simulink model "TCS1"  (R2024b)
settings: Solver=ode45  StartTime=0.0  StopTime=20  RelTol=1e-3
InitFcn:
  | Cte_TP_ABS_CHERIF
values from neighbouring files (symbols this model uses):
  g = 9.81    [Cte_TP_ABS_CHERIF.m]    (also in Cte_Traction.m)
  m = 1000    [Cte_TP_ABS_CHERIF.m]    (also in Cte_Traction.m = 1500)
  rRoue = 0.3    [Cte_TP_ABS_CHERIF.m]
libraries: simulink x4
settings Model: Creator=enzoc  LastModifiedBy=enzoc
settings SolverCC: ZeroCrossAlgorithm=Adaptive
settings DebuggingCC: IgnoredZcDiagnostic=none

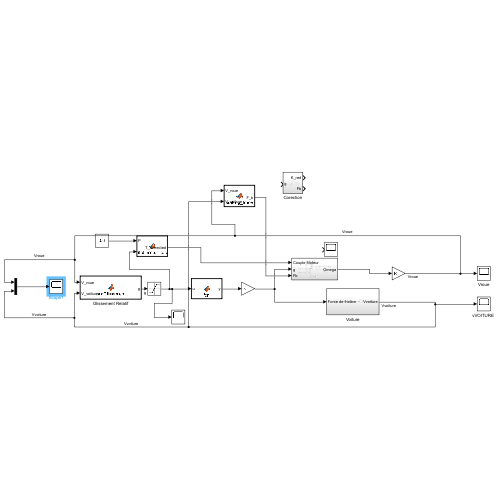
[thumbnail: Simulink's stored preview of the top-level diagram]
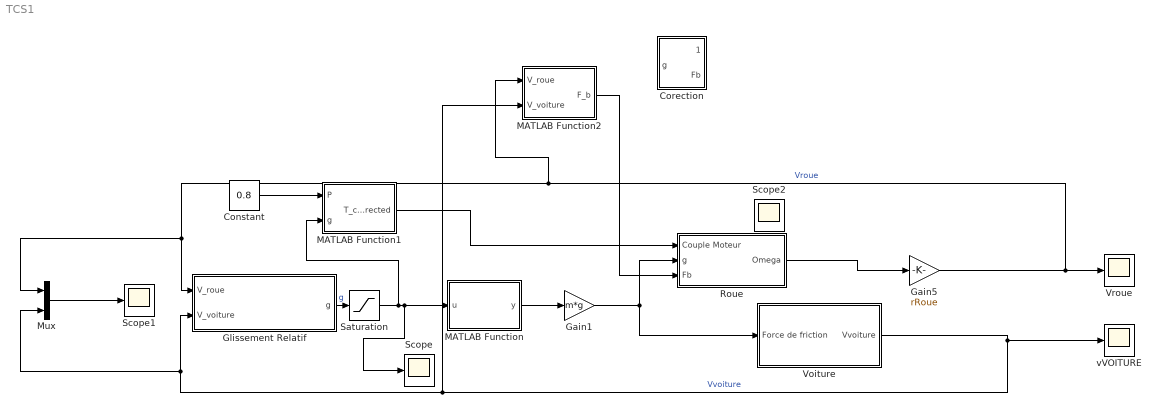
== system TCS1 ==
  Constant : Constant  Value=0.8
  Corection : Subsystem
  Gain1 : Gain  Gain=m*g
  Gain5 : Gain  Gain=rRoue
  Glissement Relatif : MATLAB Function  TreatAsAtomicUnit=on
  MATLAB Function : MATLAB Function  TreatAsAtomicUnit=on
  MATLAB Function1 : MATLAB Function  TreatAsAtomicUnit=on
  MATLAB Function2 : MATLAB Function  TreatAsAtomicUnit=on
  Mux : Mux  Inputs=2
  Roue : Subsystem
  Saturation : Saturate  UpperLimit=1  LowerLimit=-1
  Scope : Scope
  Scope1 : Scope
  Scope2 : Scope
  Voiture : Subsystem
  Vroue : Scope
  "vVOITURE " : Scope
  wires:
  Gain5/1 -> Mux/1, Glissement Relatif/1(V_roue), MATLAB Function2/1(V_roue), Vroue/1  "Vroue"
  Roue/1(Omega) -> Gain5/1
  Voiture/1(Vvoiture) -> MATLAB Function2/2(V_voiture), Mux/2, Glissement Relatif/2(V_voiture), "vVOITURE "/1  "Vvoiture"
  Mux/1 -> Scope1/1
  MATLAB Function/1(y) -> Gain1/1
  Glissement Relatif/1(g) -> Saturation/1  "g"
  Saturation/1 -> MATLAB Function1/2(g), MATLAB Function/1(u), Scope/1
  Gain1/1 -> Roue/2(g), Voiture/1(Force de friction)
  MATLAB Function2/1(F_b) -> Roue/3(Fb)
  MATLAB Function1/1(T_corrected) -> Roue/1(Couple Moteur)
  Constant/1 -> MATLAB Function1/1(P)

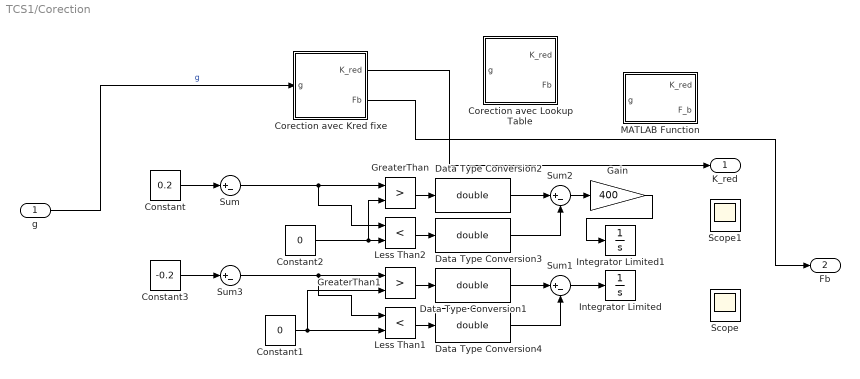
== system TCS1/Corection ==
  g : Inport
  Constant : Constant  Value=0.2
  Constant1 : Constant  Value=0
  Constant2 : Constant  Value=0
  Constant3 : Constant  Value=-0.2
  Corection avec Kred fixe : Subsystem
  Corection avec Lookup Table : Subsystem
  Data Type Conversion{1..4} (4 alike) : DataTypeConversion  OutDataTypeStr=double  SaturateOnIntegerOverflow=off
  Gain : Gain  Gain=400
  GreaterThan : RelationalOperator  Operator=>  OutDataTypeStr=boolean  RndMeth=Simplest  InputSameDT=off
  GreaterThan1 : RelationalOperator  Operator=>  OutDataTypeStr=boolean  RndMeth=Simplest  InputSameDT=off
  Integrator Limited : Integrator  LimitOutput=on  UpperSaturationLimit=1  LowerSaturationLimit=0
  Integrator Limited1 : Integrator  LimitOutput=on  UpperSaturationLimit=1  LowerSaturationLimit=0
  Less Than1 : RelationalOperator  Operator=<  OutDataTypeStr=boolean  RndMeth=Simplest  InputSameDT=off
  Less Than2 : RelationalOperator  Operator=<  OutDataTypeStr=boolean  RndMeth=Simplest  InputSameDT=off
  MATLAB Function : MATLAB Function  TreatAsAtomicUnit=on
  Scope : Scope
  Scope1 : Scope
  Sum{,1..3} (4 alike) : Sum  Inputs=|+-
  K_red : Outport
  Fb : Outport  Port=2
  wires:
  Constant/1 -> Sum/1
  Constant2/1 -> Less Than2/2, GreaterThan/2
  GreaterThan/1 -> Data Type Conversion2/1
  Sum2/1 -> Gain/1
  Data Type Conversion3/1 -> Sum2/2
  Sum/1 -> GreaterThan/1, Less Than2/1
  Less Than2/1 -> Data Type Conversion3/1
  Data Type Conversion2/1 -> Sum2/1
  Gain/1 -> Integrator Limited1/1
  Sum3/1 -> GreaterThan1/1, Less Than1/1
  Constant1/1 -> Less Than1/2, GreaterThan1/2
  Less Than1/1 -> Data Type Conversion4/1
  Data Type Conversion4/1 -> Sum1/2
  GreaterThan1/1 -> Data Type Conversion1/1
  Data Type Conversion1/1 -> Sum1/1
  Constant3/1 -> Sum3/1
  Sum1/1 -> Integrator Limited/1
  Corection avec Kred fixe/2(Fb) -> Fb/1
  Corection avec Kred fixe/1(K_red) -> K_red/1
  g/1 -> Corection avec Kred fixe/1(g)  "g"

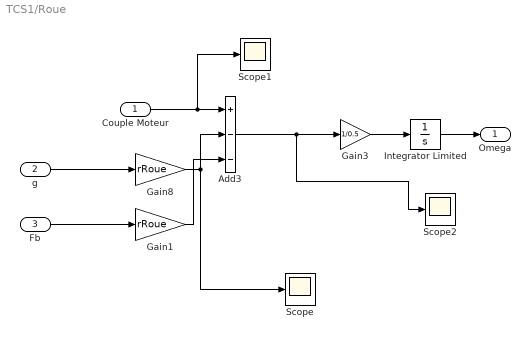
== system TCS1/Roue ==
  Couple Moteur : Inport
  g : Inport  Port=2
  Fb : Inport  Port=3
  Add3 : Sum  Inputs=+--
  Gain1 : Gain  Gain=rRoue
  Gain3 : Gain  Gain=1/0.5
  Gain8 : Gain  Gain=rRoue
  Integrator Limited : Integrator  LimitOutput=on  UpperSaturationLimit=1000  LowerSaturationLimit=0
  Scope : Scope
  Scope1 : Scope
  Scope2 : Scope
  Omega : Outport
  wires:
  Couple Moteur/1 -> Scope1/1, Add3/1
  g/1 -> Gain8/1
  Gain8/1 -> Scope/1, Add3/2
  Add3/1 -> Scope2/1, Gain3/1
  Gain3/1 -> Integrator Limited/1
  Integrator Limited/1 -> Omega/1
  Fb/1 -> Gain1/1
  Gain1/1 -> Add3/3

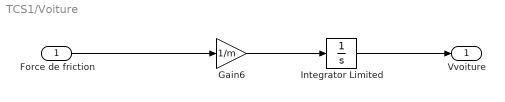
== system TCS1/Voiture ==
  Force de friction : Inport
  Gain6 : Gain  Gain=1/m
  Integrator Limited : Integrator  LimitOutput=on  UpperSaturationLimit=+inf  LowerSaturationLimit=0
  Vvoiture : Outport
  wires:
  Gain6/1 -> Integrator Limited/1
  Integrator Limited/1 -> Vvoiture/1
  Force de friction/1 -> Gain6/1

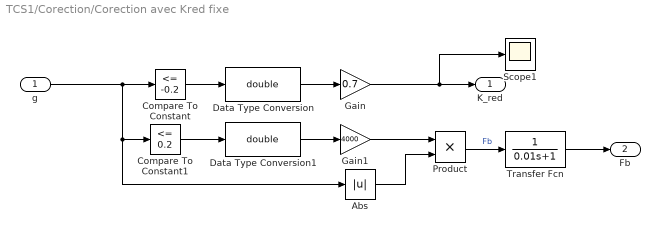
== system TCS1/Corection/Corection avec Kred fixe ==
  g : Inport
  Abs : Abs  SaturateOnIntegerOverflow=off
  Compare To Constant : simulink/Logic and Bit Operations/Compare To Constant  relop=<=  const=-0.2  OutDataTypeStr=boolean
  Compare To Constant1 : simulink/Logic and Bit Operations/Compare To Constant  relop=<=  const=0.2  OutDataTypeStr=boolean
  Data Type Conversion : DataTypeConversion  OutDataTypeStr=double  SaturateOnIntegerOverflow=off  RndMeth=Floor
  Data Type Conversion1 : DataTypeConversion  OutDataTypeStr=double  SaturateOnIntegerOverflow=off  RndMeth=Floor
  Gain : Gain  Gain=0.7
  Gain1 : Gain  Gain=4000
  Product : Product
  Scope1 : Scope
  Transfer Fcn : TransferFcn  Denominator=[0.01 1]
  K_red : Outport
  Fb : Outport  Port=2
  wires:
  g/1 -> Abs/1, Compare To Constant1/1, Compare To Constant/1
  Product/1 -> Transfer Fcn/1  "Fb"
  Abs/1 -> Product/2
  Data Type Conversion1/1 -> Gain1/1
  Compare To Constant/1 -> Data Type Conversion/1
  Compare To Constant1/1 -> Data Type Conversion1/1
  Gain1/1 -> Product/1
  Transfer Fcn/1 -> Fb/1
  Data Type Conversion/1 -> Gain/1
  Gain/1 -> Scope1/1, K_red/1

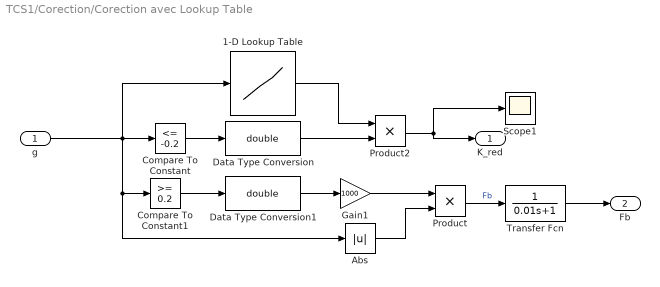
== system TCS1/Corection/Corection avec Lookup Table ==
  g : Inport
  1-D Lookup Table : Lookup_n-D  NumberOfTableDimensions=1  BreakpointsForDimension1=[-1.0, -0.9, -0.8, -0.7, -0.6, -0.5, -0.4, -0.3, -0.2, 0]  Table=[0.1, 0.15, 0.25, 0.35, 0.45, 0.55, 0.65, 0.75, 0.85, 1.0]  InternalRulePriority=Speed  RndMeth=Simplest
  Abs : Abs  SaturateOnIntegerOverflow=off
  Compare To Constant : simulink/Logic and Bit Operations/Compare To Constant  relop=<=  const=-0.2  OutDataTypeStr=boolean
  Compare To Constant1 : simulink/Logic and Bit Operations/Compare To Constant  relop=>=  const=0.2  OutDataTypeStr=boolean
  Data Type Conversion : DataTypeConversion  OutDataTypeStr=double  SaturateOnIntegerOverflow=off  RndMeth=Floor
  Data Type Conversion1 : DataTypeConversion  OutDataTypeStr=double  SaturateOnIntegerOverflow=off  RndMeth=Floor
  Gain1 : Gain  Gain=1000
  Product : Product
  Product2 : Product
  Scope1 : Scope
  Transfer Fcn : TransferFcn  Denominator=[0.01 1]
  K_red : Outport
  Fb : Outport  Port=2
  wires:
  g/1 -> 1-D Lookup Table/1, Abs/1, Compare To Constant1/1, Compare To Constant/1
  Product/1 -> Transfer Fcn/1  "Fb"
  Abs/1 -> Product/2
  Data Type Conversion1/1 -> Gain1/1
  Compare To Constant/1 -> Data Type Conversion/1
  Compare To Constant1/1 -> Data Type Conversion1/1
  Data Type Conversion/1 -> Product2/2
  Gain1/1 -> Product/1
  1-D Lookup Table/1 -> Product2/1
  Product2/1 -> K_red/1, Scope1/1
  Transfer Fcn/1 -> Fb/1

== matlab function TCS1/Corection/MATLAB Function ==
  data: g input; K_red output; F_b output
function [K_red, F_b] = traction_control(g)
    % Paramètres
    g_seuil_haut = 0.2;  % Seuil supérieur de glissement
    g_seuil_bas = -0.2;  % Seuil inférieur de glissement
    K_frein = 1000;      % Gain pour la force de freinage
    
    % Lookup Table pour K_red
    g_points = [-1, -0.9, -0.8, -0.7, -0.6, -0.5, -0.4, -0.3, -0.2, 0];
    K_red_points = [0.1, 0.15, 0.25, 0.35, 0.45, 0.55, 0.65, 0.75, 0.85, 1.0];
    
    % Initialisation des sorties
    K_red = 1.0;  % Par défaut, pas de réduction
    F_b = 0;      % Pas de freinage par défaut
    
    % Logique de contrôle pour K_red
    if g <= g_seuil_bas
        % Interpolation pour K_red en fonction de g
        K_red = interp1(g_points, K_red_points, g, 'linear', 'extrap');
    end
    
    % Logique de contrôle pour F_b
    if g > g_seuil_haut
        % Appliquer un freinage proportionnel au glissement positif excessif
        F_b = K_frein * abs(g);
    end
end

== matlab function TCS1/MATLAB Function ==
  data: u input; y output
function y = fcn(u)

y = u;

== matlab function TCS1/MATLAB Function1 ==
  data: P input; T_corrected output; g input
function T_corrected = correct_motor_torque(P, g)
    % Function to correct the motor torque based on pedal input and slip ratio
    % All parameters are defined internally.
    %
    % Inputs:
    %   P - Pedal position (0 to 1)
    %   g - Current slip ratio (dimensionless)
    %
    % Output:
    %   T_corrected - Corrected motor torque (N.m)

    % Internal parameters
    g_cible = 0.2;          % Target slip ratio
    a_max = 5;              % Maximum acceleration (m/s^2)
    m = 1500;               % Mass of the vehicle (kg)
    R_w = 0.3;              % Wheel radius (m)
    Kp = 2;                 % Proportional gain for slip correction
    T_min = 0;              % Minimum allowable torque (N.m)
    T_max = 500;            % Maximum allowable torque (N.m)

    % Step 1: Translate pedal input into desired acceleration
    a_demandee = P * a_max;  % Desired acceleration (m/s^2)

    % Step 2: Calculate the demanded torque
    T_demandee = m * a_demandee * R_w;

    % Step 3: Check if slip correction is needed
    if g > g_cible
        % Calculate the slip error
        e_g = g - g_cible;

        % Apply proportional correction to the torque
        T_corrected = T_demandee * (1 - Kp * e_g);
    else
        % No correction needed, use the demanded torque
        T_corrected = T_demandee;
    end

    % Step 4: Saturate the corrected torque to stay within limits
    T_corrected = max(T_min, min(T_max, T_corrected));
end

== matlab function TCS1/MATLAB Function2 ==
  data: V_roue input; F_b output; V_voiture input
function F_b = braking_force(V_roue, V_voiture)
    % Compute braking torque based on the slip
    %
    % Inputs:
    %   V_roue    - Speed of the wheel (rad/s or m/s)
    %   V_voiture - Speed of the vehicle (rad/s or m/s)
    %   R_w       - Wheel radius (m)
    %
    % Output:
    %   T_b - Braking torque (N.m)

    % Braking gain (K_f) - Tuning parameter
    K_f = 0;  % Adjust this value as needed for your system

    % Compute the force of braking
    F_b = K_f * (V_roue - V_voiture);
end

== matlab function TCS1/Glissement Relatif ==
  data: V_roue input; V_voiture input; g output
function g = calcGlissement(V_roue, V_voiture)
    g = (V_roue-V_voiture)/(abs(V_voiture)+0.001);
end
